simulink model "fft_overlap_tomori"  (R2023b)
settings: Solver=VariableStepAuto  StartTime=0.0  StopTime=inf  RelTol=1e-3
InitFcn:
  | fftparrallelout
  | load('dataram.mat')
  | s= fi(exp(-1j*2*pi.*(0:63)/64),1,16,15);
  | fixed_point = fixdt(1,27,20);
  | fixed_pointu = fixdt(0,29,20);
  | fixed = fixdt(1,22,15);
  | const = fixdt(1,18,17);
  | addConst = fixdt(1,18,16);
  | f =10.4e6;
  | f1=45e6;
  | alpha1 =5;
  | beta1 = 0.00001 ;
  | beta2 = 0.99999 ;
  | beta3 = 23;
undefined symbols (not defined in the file or in its folder): j
libraries: dspxfrm3 x11, commrflib2 x4
(part 2 of 10)

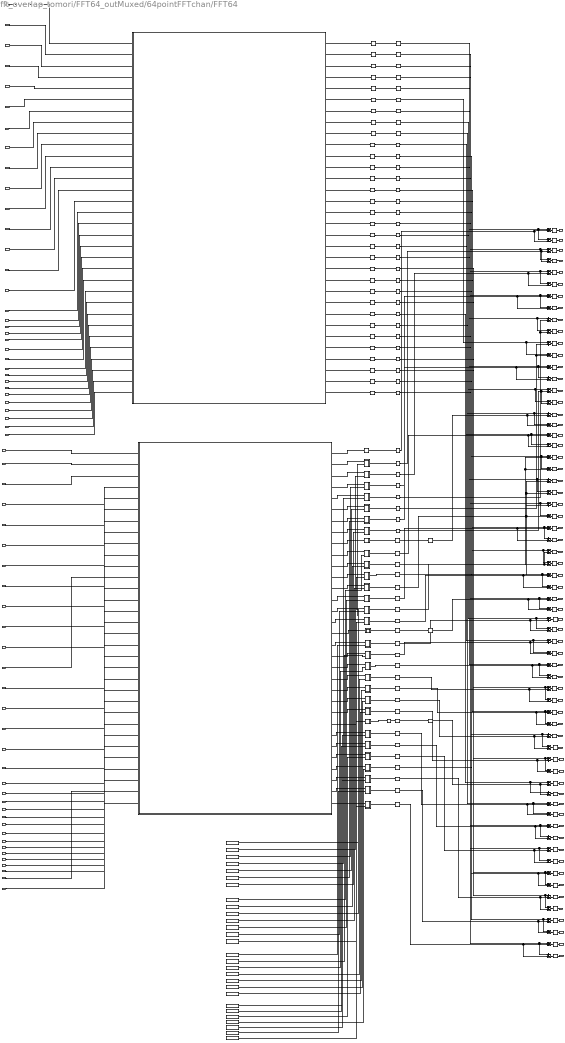
== system fft_overlap_tomori/FFT64_outMuxed/64pointFFTchan/FFT64 ==
  In1 : Inport
  In2 : Inport  Port=2
  In3 : Inport  Port=3
  In4 : Inport  Port=4
  In5 : Inport  Port=5
  In6 : Inport  Port=6
  In7 : Inport  Port=7
  In8 : Inport  Port=8
  In9 : Inport  Port=9
  In10 : Inport  Port=10
  In11 : Inport  Port=11
  In12 : Inport  Port=12
  In13 : Inport  Port=13
  In14 : Inport  Port=14
  In15 : Inport  Port=15
  In17 : Inport  Port=16
  In19 : Inport  Port=17
  In16 : Inport  Port=18
  In18 : Inport  Port=19
  In20 : Inport  Port=20
  In21 : Inport  Port=21
  In22 : Inport  Port=22
  In23 : Inport  Port=23
  In24 : Inport  Port=24
  In25 : Inport  Port=25
  In26 : Inport  Port=26
  In27 : Inport  Port=27
  In28 : Inport  Port=28
  In29 : Inport  Port=29
  In30 : Inport  Port=30
  In31 : Inport  Port=31
  In32 : Inport  Port=32
  In33 : Inport  Port=33
  In34 : Inport  Port=34
  In35 : Inport  Port=35
  In36 : Inport  Port=36
  In37 : Inport  Port=37
  In38 : Inport  Port=38
  In39 : Inport  Port=39
  In40 : Inport  Port=40
  In41 : Inport  Port=41
  In42 : Inport  Port=42
  In43 : Inport  Port=43
  In44 : Inport  Port=44
  In45 : Inport  Port=45
  In46 : Inport  Port=46
  In47 : Inport  Port=47
  In48 : Inport  Port=48
  In49 : Inport  Port=49
  In50 : Inport  Port=50
  In51 : Inport  Port=51
  In52 : Inport  Port=52
  In53 : Inport  Port=53
  In54 : Inport  Port=54
  In55 : Inport  Port=55
  In56 : Inport  Port=56
  In57 : Inport  Port=57
  In58 : Inport  Port=58
  In59 : Inport  Port=59
  In60 : Inport  Port=60
  In61 : Inport  Port=61
  In62 : Inport  Port=62
  In63 : Inport  Port=63
  In64 : Inport  Port=64
  Add{,2,4,6,8,10,12,14,16,18,20,22,24,26,28,30,32,34,36,38,40,42,44..45,47,49,51,53,56,58,60,62} (32 alike) : Sum  OutDataTypeStr=fixed  RndMeth=Round
  Add{1,3,5,7,9,11,13,15,17,19,21,23,25,27,29,31,33,35,37,39,41,43,46,48,50,52,54..55,57,59,61,63} (32 alike) : Sum  Inputs=+-  OutDataTypeStr=fixed  RndMeth=Round
  Constant1 : Constant  Value=exp(-1j*pi/8)  OutDataTypeStr=const  SampleTime=-1
  Constant10 : Constant  Value=exp(-1j*pi*13/16)  OutDataTypeStr=const  SampleTime=-1
  Constant11 : Constant  Value=exp(-1j*pi/32)  OutDataTypeStr=const  SampleTime=-1
  Constant12 : Constant  Value=exp(-1j*7*pi/8)  OutDataTypeStr=const  SampleTime=-1
  Constant13 : Constant  Value=exp(-1j*pi*15/16)  OutDataTypeStr=const  SampleTime=-1
  Constant14 : Constant  Value=exp(-1j*3*pi/32)  OutDataTypeStr=const  SampleTime=-1
  Constant15 : Constant  Value=exp(-1j*pi*3/16)  OutDataTypeStr=const  SampleTime=-1
  Constant16 : Constant  Value=exp(-1j*pi*7/32)  OutDataTypeStr=const  SampleTime=-1
  Constant17 : Constant  Value=exp(-1j*pi*9/32)  OutDataTypeStr=const  SampleTime=-1
  Constant18 : Constant  Value=exp(-1j*pi*11/32)  OutDataTypeStr=const  SampleTime=-1
  Constant19 : Constant  Value=exp(-1j*pi*13/32)  OutDataTypeStr=const  SampleTime=-1
  Constant2 : Constant  Value=exp(-1j*pi/16)  OutDataTypeStr=const  SampleTime=-1
  Constant20 : Constant  Value=exp(-1j*pi*15/32)  OutDataTypeStr=const  SampleTime=-1
  Constant21 : Constant  Value=exp(-1j*pi*17/32)  OutDataTypeStr=const  SampleTime=-1
  Constant22 : Constant  Value=exp(-1j*pi*19/32)  OutDataTypeStr=const  SampleTime=-1
  Constant23 : Constant  Value=exp(-1j*pi*21/32)  OutDataTypeStr=const  SampleTime=-1
  Constant24 : Constant  Value=exp(-1j*pi*23/32)  OutDataTypeStr=const  SampleTime=-1
  Constant25 : Constant  Value=exp(-1j*pi*25/32)  OutDataTypeStr=const  SampleTime=-1
  Constant26 : Constant  Value=exp(-1j*pi*27/32)  OutDataTypeStr=const  SampleTime=-1
  Constant27 : Constant  Value=exp(-1j*pi*29/32)  OutDataTypeStr=const  SampleTime=-1
  Constant28 : Constant  Value=exp(-1j*pi*31/32)  OutDataTypeStr=const  SampleTime=-1
  Constant3 : Constant  Value=exp(-1j*pi*5/32)  OutDataTypeStr=const  SampleTime=-1
  Constant4 : Constant  Value=exp(-1j*pi*5/16)  OutDataTypeStr=const  SampleTime=-1
  Constant5 : Constant  Value=exp(-1j*pi*3/8)  OutDataTypeStr=const  SampleTime=-1
  Constant6 : Constant  Value=exp(-1j*pi*5/8)  OutDataTypeStr=const  SampleTime=-1
  Constant7 : Constant  Value=exp(-1j*pi*7/16)  OutDataTypeStr=const  SampleTime=-1
  Constant8 : Constant  Value=exp(-1j*pi*9/16)  OutDataTypeStr=const  SampleTime=-1
  Constant9 : Constant  Value=exp(-1j*pi*11/16)  OutDataTypeStr=const  SampleTime=-1
  Delay{,9..15,17,20..21,27..32,50..51,53..59,61..98,133..147,149..163} (94 alike) : Delay  DelayLength=1
  Delay{1..8,16,18..19,22..26,33..49,52,60,99..132,164} (70 alike) : Delay  DelayLength=3
  FFT32 : Subsystem
  FFT32_1 : Subsystem
  complexmult : Subsystem
  complexmult1 : Subsystem
  complexmult10 : Subsystem
  complexmult11 : Subsystem
  complexmult12 : Subsystem
  complexmult13 : Subsystem
  complexmult14 : Subsystem
  complexmult15 : Subsystem
  complexmult16 : Subsystem
  complexmult17 : Subsystem
  complexmult18 : Subsystem
  complexmult19 : Subsystem
  complexmult2 : Subsystem
  complexmult20 : Subsystem
  complexmult21 : Subsystem
  complexmult22 : Subsystem
  complexmult23 : Subsystem
  complexmult24 : Subsystem
  complexmult25 : Subsystem
  complexmult26 : Subsystem
  complexmult27 : Subsystem
  complexmult3 : Subsystem
  complexmult4 : Subsystem
  complexmult5 : Subsystem
  complexmult6 : Subsystem
  complexmult7 : Subsystem
  complexmult8 : Subsystem
  complexmult9 : Subsystem
  multByExp(-j*Pi/4) : Subsystem
  multByExp(-j*Pi/4)1 : Subsystem
  multByMinusJ : Subsystem
  multByMinusJ3 : Subsystem
  Out1 : Outport  VectorParamsAs1DForOutWhenUnconnected=off
  Out2 : Outport  Port=2  VectorParamsAs1DForOutWhenUnconnected=off
  Out4 : Outport  Port=3  VectorParamsAs1DForOutWhenUnconnected=off
  Out3 : Outport  Port=4  VectorParamsAs1DForOutWhenUnconnected=off
  Out5 : Outport  Port=5  VectorParamsAs1DForOutWhenUnconnected=off
  Out6 : Outport  Port=6  VectorParamsAs1DForOutWhenUnconnected=off
  Out7 : Outport  Port=7  VectorParamsAs1DForOutWhenUnconnected=off
  Out8 : Outport  Port=8  VectorParamsAs1DForOutWhenUnconnected=off
  Out9 : Outport  Port=9  VectorParamsAs1DForOutWhenUnconnected=off
  Out10 : Outport  Port=10  VectorParamsAs1DForOutWhenUnconnected=off
  Out11 : Outport  Port=11  VectorParamsAs1DForOutWhenUnconnected=off
  Out12 : Outport  Port=12  VectorParamsAs1DForOutWhenUnconnected=off
  Out13 : Outport  Port=13  VectorParamsAs1DForOutWhenUnconnected=off
  Out14 : Outport  Port=14  VectorParamsAs1DForOutWhenUnconnected=off
  Out15 : Outport  Port=15  VectorParamsAs1DForOutWhenUnconnected=off
  Out16 : Outport  Port=16  VectorParamsAs1DForOutWhenUnconnected=off
  Out17 : Outport  Port=17  VectorParamsAs1DForOutWhenUnconnected=off
  Out18 : Outport  Port=18  VectorParamsAs1DForOutWhenUnconnected=off
  Out19 : Outport  Port=19  VectorParamsAs1DForOutWhenUnconnected=off
  Out20 : Outport  Port=20  VectorParamsAs1DForOutWhenUnconnected=off
  Out21 : Outport  Port=21  VectorParamsAs1DForOutWhenUnconnected=off
  Out22 : Outport  Port=22  VectorParamsAs1DForOutWhenUnconnected=off
  Out23 : Outport  Port=23  VectorParamsAs1DForOutWhenUnconnected=off
  Out24 : Outport  Port=24  VectorParamsAs1DForOutWhenUnconnected=off
  Out25 : Outport  Port=25  VectorParamsAs1DForOutWhenUnconnected=off
  Out26 : Outport  Port=26  VectorParamsAs1DForOutWhenUnconnected=off
  Out27 : Outport  Port=27  VectorParamsAs1DForOutWhenUnconnected=off
  Out28 : Outport  Port=28  VectorParamsAs1DForOutWhenUnconnected=off
  Out29 : Outport  Port=29  VectorParamsAs1DForOutWhenUnconnected=off
  Out30 : Outport  Port=30  VectorParamsAs1DForOutWhenUnconnected=off
  Out31 : Outport  Port=31  VectorParamsAs1DForOutWhenUnconnected=off
  Out32 : Outport  Port=32  VectorParamsAs1DForOutWhenUnconnected=off
  Out33 : Outport  Port=33  VectorParamsAs1DForOutWhenUnconnected=off
  Out34 : Outport  Port=34  VectorParamsAs1DForOutWhenUnconnected=off
  Out35 : Outport  Port=35  VectorParamsAs1DForOutWhenUnconnected=off
  Out36 : Outport  Port=36  VectorParamsAs1DForOutWhenUnconnected=off
  Out37 : Outport  Port=37  VectorParamsAs1DForOutWhenUnconnected=off
  Out38 : Outport  Port=38  VectorParamsAs1DForOutWhenUnconnected=off
  Out39 : Outport  Port=39  VectorParamsAs1DForOutWhenUnconnected=off
  Out40 : Outport  Port=40  VectorParamsAs1DForOutWhenUnconnected=off
  Out41 : Outport  Port=41  VectorParamsAs1DForOutWhenUnconnected=off
  Out42 : Outport  Port=42  VectorParamsAs1DForOutWhenUnconnected=off
  Out43 : Outport  Port=43  VectorParamsAs1DForOutWhenUnconnected=off
  Out44 : Outport  Port=44  VectorParamsAs1DForOutWhenUnconnected=off
  Out45 : Outport  Port=45  VectorParamsAs1DForOutWhenUnconnected=off
  Out46 : Outport  Port=46  VectorParamsAs1DForOutWhenUnconnected=off
  Out47 : Outport  Port=47  VectorParamsAs1DForOutWhenUnconnected=off
  Out48 : Outport  Port=48  VectorParamsAs1DForOutWhenUnconnected=off
  Out49 : Outport  Port=49  VectorParamsAs1DForOutWhenUnconnected=off
  Out50 : Outport  Port=50  VectorParamsAs1DForOutWhenUnconnected=off
  Out51 : Outport  Port=51  VectorParamsAs1DForOutWhenUnconnected=off
  Out52 : Outport  Port=52  VectorParamsAs1DForOutWhenUnconnected=off
  Out53 : Outport  Port=53  VectorParamsAs1DForOutWhenUnconnected=off
  Out54 : Outport  Port=54  VectorParamsAs1DForOutWhenUnconnected=off
  Out55 : Outport  Port=55  VectorParamsAs1DForOutWhenUnconnected=off
  Out56 : Outport  Port=56  VectorParamsAs1DForOutWhenUnconnected=off
  Out57 : Outport  Port=57  VectorParamsAs1DForOutWhenUnconnected=off
  Out58 : Outport  Port=58  VectorParamsAs1DForOutWhenUnconnected=off
  Out59 : Outport  Port=59  VectorParamsAs1DForOutWhenUnconnected=off
  Out60 : Outport  Port=60  VectorParamsAs1DForOutWhenUnconnected=off
  Out61 : Outport  Port=61  VectorParamsAs1DForOutWhenUnconnected=off
  Out62 : Outport  Port=62  VectorParamsAs1DForOutWhenUnconnected=off
  Out63 : Outport  Port=63  VectorParamsAs1DForOutWhenUnconnected=off
  Out64 : Outport  Port=64  VectorParamsAs1DForOutWhenUnconnected=off
  wires:
  In13/1 -> FFT32/7(In7)
  In15/1 -> FFT32/8(In8)
  In11/1 -> FFT32/6(In6)
  In19/1 -> FFT32/9(In9)
  In9/1 -> FFT32/5(In5)
  In18/1 -> FFT32/10(In10)
  In7/1 -> FFT32/4(In4)
  In21/1 -> FFT32/11(In11)
  In5/1 -> FFT32/3(In3)
  In23/1 -> FFT32/12(In12)
  In3/1 -> FFT32/2(In2)
  In25/1 -> FFT32/13(In13)
  In1/1 -> FFT32/1(In1)
  In27/1 -> FFT32/14(In14)
  In29/1 -> FFT32/15(In15)
  In31/1 -> FFT32/16(In17)
  In33/1 -> FFT32/17(In19)
  In63/1 -> FFT32/32(In32)
  In61/1 -> FFT32/31(In31)
  In59/1 -> FFT32/30(In30)
  In57/1 -> FFT32/29(In29)
  In55/1 -> FFT32/28(In28)
  In53/1 -> FFT32/27(In27)
  In51/1 -> FFT32/26(In26)
  In49/1 -> FFT32/25(In25)
  In47/1 -> FFT32/24(In24)
  In45/1 -> FFT32/23(In23)
  In43/1 -> FFT32/22(In22)
  In41/1 -> FFT32/21(In21)
  In39/1 -> FFT32/20(In20)
  In37/1 -> FFT32/19(In18)
  In35/1 -> FFT32/18(In16)
  In12/1 -> FFT32_1/6(In6)
  In14/1 -> FFT32_1/7(In7)
  In10/1 -> FFT32_1/5(In5)
  In17/1 -> FFT32_1/8(In8)
  In8/1 -> FFT32_1/4(In4)
  In16/1 -> FFT32_1/9(In9)
  In6/1 -> FFT32_1/3(In3)
  In20/1 -> FFT32_1/10(In10)
  In4/1 -> FFT32_1/2(In2)
  In2/1 -> FFT32_1/1(In1)
  In22/1 -> FFT32_1/11(In11)
  In64/1 -> FFT32_1/32(In32)
  In62/1 -> FFT32_1/31(In31)
  In24/1 -> FFT32_1/12(In12)
  In60/1 -> FFT32_1/30(In30)
  In58/1 -> FFT32_1/29(In29)
  In26/1 -> FFT32_1/13(In13)
  In56/1 -> FFT32_1/28(In28)
  In54/1 -> FFT32_1/27(In27)
  In28/1 -> FFT32_1/14(In14)
  In52/1 -> FFT32_1/26(In26)
  In50/1 -> FFT32_1/25(In25)
  In30/1 -> FFT32_1/15(In15)
  In48/1 -> FFT32_1/24(In24)
  In46/1 -> FFT32_1/23(In23)
  In44/1 -> FFT32_1/22(In22)
  In32/1 -> FFT32_1/16(In17)
  In42/1 -> FFT32_1/21(In21)
  In40/1 -> FFT32_1/20(In20)
  In34/1 -> FFT32_1/17(In19)
  In38/1 -> FFT32_1/19(In18)
  In36/1 -> FFT32_1/18(In16)
  FFT32/1(x0) -> Delay22/1
  FFT32/2(x1) -> Delay18/1
  FFT32/3(x2) -> Delay19/1
  FFT32/4(x3) -> Delay16/1
  FFT32/5(x4) -> Delay23/1
  FFT32/6(x5) -> Delay24/1
  FFT32/7(x6) -> Delay26/1
  FFT32/8(x7) -> Delay33/1
  FFT32/9(x8) -> Delay34/1
  FFT32/10(x9) -> Delay35/1
  FFT32/11(x10) -> Delay37/1
  FFT32/12(x11) -> Delay38/1
  FFT32/13(x12) -> Delay39/1
  FFT32/14(x13) -> Delay36/1
  FFT32/15(x14) -> Delay40/1
  FFT32/16(x15) -> Delay41/1
  FFT32/17(x16) -> Delay42/1
  FFT32/18(x17) -> Delay43/1
  FFT32/19(x18) -> Delay44/1
  FFT32/20(x19) -> Delay45/1
  FFT32/21(x20) -> Delay46/1
  FFT32/22(x21) -> Delay47/1
  FFT32/23(x22) -> Delay48/1
  FFT32/24(x23) -> Delay49/1
  FFT32/25(x24) -> Delay1/1
  FFT32/26(x25) -> Delay2/1
  FFT32/27(x26) -> Delay3/1
  FFT32/28(x27) -> Delay4/1
  FFT32/29(x28) -> Delay5/1
  FFT32/30(x29) -> Delay6/1
  FFT32/31(x30) -> Delay7/1
  FFT32/32(x31) -> Delay8/1
  FFT32_1/25(x24) -> multByExp(-j*Pi/4)1/1(x4)
  Delay22/1 -> Delay105/1
  Delay18/1 -> Delay102/1
  Delay19/1 -> Delay103/1
  Delay16/1 -> Delay101/1
  Delay23/1 -> Delay106/1
  Delay24/1 -> Delay107/1
  Delay26/1 -> Delay108/1
  Delay33/1 -> Delay110/1
  Delay34/1 -> Delay111/1
  Delay35/1 -> Delay112/1
  Delay37/1 -> Delay114/1
  Delay38/1 -> Delay115/1
  Delay39/1 -> Delay116/1
  Delay36/1 -> Delay113/1
  Delay40/1 -> Delay118/1
  Delay41/1 -> Delay119/1
  Delay42/1 -> Delay120/1
  Delay43/1 -> Delay121/1
  Delay44/1 -> Delay122/1
  Delay45/1 -> Delay123/1
  Delay46/1 -> Delay124/1
  Delay47/1 -> Delay125/1
  Delay48/1 -> Delay126/1
  Delay49/1 -> Delay127/1
  Delay1/1 -> Delay100/1
  Delay2/1 -> Delay104/1
  Delay3/1 -> Delay109/1
  Delay4/1 -> Delay117/1
  Delay5/1 -> Delay128/1
  Delay6/1 -> Delay129/1
  Delay7/1 -> Delay130/1
  Delay8/1 -> Delay131/1
  FFT32_1/1(x0) -> Delay99/1
  Add4/1 -> Delay17/1
  Add/1 -> Delay/1
  Add2/1 -> Delay66/1
  Add6/1 -> Delay20/1
  Add8/1 -> Delay21/1
  Add10/1 -> Delay9/1
  Add12/1 -> Delay12/1
  Add14/1 -> Delay13/1
  Add16/1 -> Delay32/1
  Add24/1 -> Delay65/1
  Add26/1 -> Delay56/1
  Add28/1 -> Delay57/1
  Add30/1 -> Delay58/1
  Add18/1 -> Delay59/1
  Add20/1 -> Delay51/1
  Add22/1 -> Delay53/1
  Add32/1 -> Delay67/1
  Add44/1 -> Delay97/1
  Add58/1 -> Delay74/1
  Add60/1 -> Delay75/1
  Add62/1 -> Delay76/1
  Add34/1 -> Delay98/1
  Add36/1 -> Delay70/1
  Add38/1 -> Delay71/1
  Add40/1 -> Delay82/1
  Add49/1 -> Delay96/1
  Add51/1 -> Delay88/1
  Add53/1 -> Delay89/1
  Add56/1 -> Delay90/1
  Add42/1 -> Delay91/1
  Add45/1 -> Delay84/1
  Add47/1 -> Delay85/1
  Add1/1 -> Delay28/1
  Add3/1 -> Delay29/1
  Add5/1 -> Delay30/1
  Add7/1 -> Delay31/1
  Add9/1 -> Delay10/1
  Add11/1 -> Delay11/1
  Add13/1 -> Delay14/1
  Add15/1 -> Delay15/1
  Add17/1 -> Delay61/1
  Add25/1 -> Delay62/1
  Add27/1 -> Delay63/1
  Add29/1 -> Delay64/1
  Add31/1 -> Delay27/1
  Add19/1 -> Delay50/1
  Add21/1 -> Delay54/1
  Add23/1 -> Delay55/1
  Add33/1 -> Delay78/1
  Add55/1 -> Delay79/1
  Add59/1 -> Delay80/1
  Add61/1 -> Delay81/1
  Add63/1 -> Delay68/1
  Add35/1 -> Delay69/1
  Add37/1 -> Delay72/1
  Add39/1 -> Delay73/1
  Add41/1 -> Delay92/1
  Add50/1 -> Delay93/1
  Add52/1 -> Delay94/1
  Add54/1 -> Delay95/1
  Add57/1 -> Delay77/1
  Add43/1 -> Delay83/1
  Add46/1 -> Delay86/1
  Add48/1 -> Delay87/1
  FFT32_1/2(x1) -> complexmult/1(x1)
  Constant11/1 -> complexmult/2(In3)
  complexmult/1(Out1) -> Delay133/1
  FFT32_1/3(x2) -> complexmult1/1(x1)
  Constant2/1 -> complexmult1/2(In3)
  FFT32_1/4(x3) -> complexmult2/1(x1)
  Constant14/1 -> complexmult2/2(In3)
  FFT32_1/5(x4) -> complexmult3/1(x1)
  Constant1/1 -> complexmult3/2(In3)
  FFT32_1/6(x5) -> complexmult4/1(x1)
  Constant3/1 -> complexmult4/2(In3)
  FFT32_1/7(x6) -> complexmult5/1(x1)
  multByExp(-j*Pi/4)/1(Out1) -> Delay140/1
  FFT32_1/10(x9) -> complexmult7/1(x1)
  Constant15/1 -> complexmult5/2(In3)
  FFT32_1/9(x8) -> multByExp(-j*Pi/4)/1(x4)
  FFT32_1/8(x7) -> complexmult6/1(x1)
  Constant16/1 -> complexmult6/2(In3)
  Constant17/1 -> complexmult7/2(In3)
  FFT32_1/11(x10) -> complexmult8/1(x1)
  Constant4/1 -> complexmult8/2(In3)
  FFT32_1/12(x11) -> complexmult9/1(x1)
  Constant18/1 -> complexmult9/2(In3)
  FFT32_1/13(x12) -> complexmult10/1(x1)
  Constant5/1 -> complexmult10/2(In3)
  FFT32_1/14(x13) -> complexmult11/1(x1)
  FFT32_1/15(x14) -> complexmult12/1(x1)
  Constant7/1 -> complexmult12/2(In3)
  FFT32_1/16(x15) -> complexmult13/1(x1)
  Constant20/1 -> complexmult13/2(In3)
  FFT32_1/17(x16) -> multByMinusJ/1(x4)
  multByMinusJ/1(Out1) -> Delay25/1
  FFT32_1/18(x17) -> complexmult14/1(x1)
  Constant21/1 -> complexmult14/2(In3)
  FFT32_1/19(x18) -> complexmult15/1(x1)
  FFT32_1/20(x19) -> complexmult16/1(x1)
  FFT32_1/21(x20) -> complexmult17/1(x1)
  FFT32_1/22(x21) -> complexmult18/1(x1)
  FFT32_1/23(x22) -> complexmult19/1(x1)
  Constant19/1 -> complexmult11/2(In3)
  Constant8/1 -> complexmult15/2(In3)
  Constant22/1 -> complexmult16/2(In3)
  Constant6/1 -> complexmult17/2(In3)
  Constant23/1 -> complexmult18/2(In3)
  Constant9/1 -> complexmult19/2(In3)
  FFT32_1/24(x23) -> complexmult20/1(x1)
  Constant24/1 -> complexmult20/2(In3)
  multByMinusJ3/1(Out1) -> Delay156/1
  multByExp(-j*Pi/4)1/1(Out1) -> multByMinusJ3/1(In1)
  FFT32_1/26(x25) -> complexmult21/1(x1)
  FFT32_1/27(x26) -> complexmult22/1(x1)
  FFT32_1/28(x27) -> complexmult23/1(x1)
  FFT32_1/29(x28) -> complexmult24/1(x1)
  FFT32_1/30(x29) -> complexmult25/1(x1)
  FFT32_1/32(x31) -> complexmult27/1(x1)
  FFT32_1/31(x30) -> complexmult26/1(x1)
  Constant25/1 -> complexmult21/2(In3)
  Constant10/1 -> complexmult22/2(In3)
  Constant26/1 -> complexmult23/2(In3)
  Constant12/1 -> complexmult24/2(In3)
  Constant27/1 -> complexmult25/2(In3)
  Constant13/1 -> complexmult26/2(In3)
  Constant28/1 -> complexmult27/2(In3)
  Delay82/1 -> Out25/1
  Delay83/1 -> Out62/1
  Delay84/1 -> Out31/1
  Delay85/1 -> Out32/1
  Delay86/1 -> Out63/1
  Delay77/1 -> Out61/1
  Delay73/1 -> Out56/1
  Delay71/1 -> Out24/1
  Delay91/1 -> Out30/1
  Delay92/1 -> Out57/1
  Delay93/1 -> Out58/1
  Delay94/1 -> Out59/1
  Delay95/1 -> Out60/1
  Delay96/1 -> Out26/1
  Delay87/1 -> Out64/1
  Delay88/1 -> Out27/1
  Delay89/1 -> Out28/1
  Delay90/1 -> Out29/1
  Delay72/1 -> Out55/1
  Delay70/1 -> Out23/1
  Delay69/1 -> Out54/1
  Delay98/1 -> Out22/1
  Delay68/1 -> Out53/1
  Delay76/1 -> Out21/1
  Delay81/1 -> Out52/1
  Delay75/1 -> Out20/1
  Delay74/1 -> Out19/1
  Delay80/1 -> Out51/1
  Delay79/1 -> Out50/1
  Delay97/1 -> Out18/1
  Delay78/1 -> Out49/1
  Delay67/1 -> Out17/1
  Delay50/1 -> Out46/1
  Delay28/1 -> Out33/1
  Delay14/1 -> Out39/1
  Delay17/1 -> Out4/1
  Delay12/1 -> Out7/1
  Delay54/1 -> Out47/1
  Delay10/1 -> Out37/1
  Delay59/1 -> Out14/1
  Delay51/1 -> Out15/1
  Delay21/1 -> Out5/1
  Delay/1 -> Out1/1
  Delay11/1 -> Out38/1
  Delay55/1 -> Out48/1
  Delay13/1 -> Out8/1
  Delay31/1 -> Out36/1
  Delay27/1 -> Out45/1
  Delay9/1 -> Out6/1
  Delay66/1 -> Out2/1
  Delay30/1 -> Out35/1
  Delay53/1 -> Out16/1
  Delay29/1 -> Out34/1
  Delay20/1 -> Out3/1
  Delay58/1 -> Out13/1
  Delay64/1 -> Out44/1
  Delay57/1 -> Out12/1
  Delay63/1 -> Out43/1
  Delay56/1 -> Out11/1
  Delay62/1 -> Out42/1
  Delay65/1 -> Out10/1
  Delay61/1 -> Out41/1
  Delay32/1 -> Out9/1
  Delay15/1 -> Out40/1
  complexmult1/1(Out1) -> Delay134/1
  complexmult2/1(Out1) -> Delay135/1
  complexmult3/1(Out1) -> Delay136/1
  complexmult4/1(Out1) -> Delay137/1
  complexmult5/1(Out1) -> Delay138/1
  complexmult6/1(Out1) -> Delay139/1
  Delay132/1 -> Add17/2, Add16/2
  complexmult7/1(Out1) -> Delay141/1
  complexmult8/1(Out1) -> Delay142/1
  complexmult9/1(Out1) -> Delay143/1
  complexmult10/1(Out1) -> Delay144/1
  complexmult11/1(Out1) -> Delay145/1
  complexmult12/1(Out1) -> Delay146/1
  complexmult13/1(Out1) -> Delay147/1
  Delay52/1 -> Add33/2, Add32/2
  complexmult14/1(Out1) -> Delay149/1
  complexmult15/1(Out1) -> Delay150/1
  complexmult16/1(Out1) -> Delay151/1
  complexmult17/1(Out1) -> Delay152/1
  complexmult18/1(Out1) -> Delay153/1
  complexmult19/1(Out1) -> Delay154/1
  complexmult20/1(Out1) -> Delay155/1
  Delay60/1 -> Add41/2, Add40/2
  complexmult21/1(Out1) -> Delay157/1
  complexmult22/1(Out1) -> Delay158/1
  complexmult23/1(Out1) -> Delay159/1
  complexmult24/1(Out1) -> Delay160/1
  complexmult25/1(Out1) -> Delay161/1
  complexmult26/1(Out1) -> Delay162/1
  complexmult27/1(Out1) -> Delay163/1
  Delay99/1 -> Delay164/1
  Delay105/1 -> Add1/1, Add/1
  Delay102/1 -> Add3/1, Add2/1
  Delay103/1 -> Add5/1, Add4/1
  Delay101/1 -> Add6/1, Add7/1
  Delay106/1 -> Add9/1, Add8/1
  Delay107/1 -> Add11/1, Add10/1
  Delay108/1 -> Add13/1, Add12/1
  Delay110/1 -> Add15/1, Add14/1
  Delay111/1 -> Add17/1, Add16/1
  Delay112/1 -> Add24/1, Add25/1
  Delay114/1 -> Add27/1, Add26/1
  Delay115/1 -> Add29/1, Add28/1
  Delay116/1 -> Add31/1, Add30/1
  Delay113/1 -> Add19/1, Add18/1
  Delay118/1 -> Add21/1, Add20/1
  Delay119/1 -> Add23/1, Add22/1
  Delay120/1 -> Add33/1, Add32/1
  Delay121/1 -> Add55/1, Add44/1
  Delay122/1 -> Add59/1, Add58/1
  Delay123/1 -> Add61/1, Add60/1
  Delay124/1 -> Add63/1, Add62/1
  Delay125/1 -> Add35/1, Add34/1
  Delay126/1 -> Add37/1, Add36/1
  Delay127/1 -> Add39/1, Add38/1
  Delay100/1 -> Add40/1, Add41/1
  Delay104/1 -> Add50/1, Add49/1
  Delay109/1 -> Add52/1, Add51/1
  Delay117/1 -> Add54/1, Add53/1
  Delay128/1 -> Add57/1, Add56/1
  Delay129/1 -> Add43/1, Add42/1
  Delay130/1 -> Add46/1, Add45/1
  Delay131/1 -> Add48/1, Add47/1
  Delay164/1 -> Add/2, Add1/2
  Delay133/1 -> Add3/2, Add2/2
  Delay134/1 -> Add5/2, Add4/2
  Delay135/1 -> Add7/2, Add6/2
  Delay136/1 -> Add8/2, Add9/2
  Delay137/1 -> Add10/2, Add11/2
  Delay138/1 -> Add13/2, Add12/2
  Delay139/1 -> Add15/2, Add14/2
  Delay140/1 -> Delay132/1
  Delay141/1 -> Add25/2, Add24/2
  Delay142/1 -> Add26/2, Add27/2
  Delay143/1 -> Add28/2, Add29/2
  Delay144/1 -> Add30/2, Add31/2
  Delay145/1 -> Add19/2, Add18/2
  Delay146/1 -> Add20/2, Add21/2
  Delay147/1 -> Add23/2, Add22/2
  Delay25/1 -> Delay52/1
  Delay149/1 -> Add55/2, Add44/2
  Delay150/1 -> Add59/2, Add58/2
  Delay151/1 -> Add61/2, Add60/2
  Delay152/1 -> Add63/2, Add62/2
  Delay153/1 -> Add35/2, Add34/2
  Delay154/1 -> Add37/2, Add36/2
  Delay155/1 -> Add39/2, Add38/2
  Delay156/1 -> Delay60/1
  Delay157/1 -> Add50/2, Add49/2
  Delay158/1 -> Add52/2, Add51/2
  Delay159/1 -> Add54/2, Add53/2
  Delay160/1 -> Add57/2, Add56/2
  Delay161/1 -> Add43/2, Add42/2
  Delay162/1 -> Add46/2, Add45/2
  Delay163/1 -> Add48/2, Add47/2

== system fft_overlap_tomori/16//32 and test junk/16/FFT16/FFT8 ==
  In1 : Inport
  In2 : Inport  Port=2
  In3 : Inport  Port=3
  In4 : Inport  Port=4
  In5 : Inport  Port=5
  In6 : Inport  Port=6
  In7 : Inport  Port=7
  In8 : Inport  Port=8
  Add{,2,4,6,8,10,12,14,16,18,20,22} (12 alike) : Sum  OutDataTypeStr=fixed  RndMeth=Round
  Add{1,3,5,7,9,11,13,15,17,19,21,23} (12 alike) : Sum  Inputs=+-  OutDataTypeStr=fixed  RndMeth=Round
  Delay{,1,4..9,12..13,16..23} (18 alike) : Delay  DelayLength=1
  Delay{2..3,10..11,14..15} (6 alike) : Delay  DelayLength=3
  multByExp(-j*Pi/4) : Subsystem
  multByExp(-j*Pi/4)1 : Subsystem
  multByMinusJ : Subsystem
  multByMinusJ1 : Subsystem
  multByMinusJ2 : Subsystem
  multByMinusJ3 : Subsystem
  x0 : Outport
  x1 : Outport  Port=2  VectorParamsAs1DForOutWhenUnconnected=off
  x2 : Outport  Port=3  VectorParamsAs1DForOutWhenUnconnected=off
  x3 : Outport  Port=4  VectorParamsAs1DForOutWhenUnconnected=off
  x4 : Outport  Port=5  VectorParamsAs1DForOutWhenUnconnected=off
  x5 : Outport  Port=6  VectorParamsAs1DForOutWhenUnconnected=off
  x6 : Outport  Port=7  VectorParamsAs1DForOutWhenUnconnected=off
  x7 : Outport  Port=8  VectorParamsAs1DForOutWhenUnconnected=off
  wires:
  In1/1 -> Add1/1, Add/1
  In5/1 -> Add/2, Add1/2
  Add/1 -> Delay/1
  Add1/1 -> Delay1/1
  Delay/1 -> Add2/1, Add3/1
  Add2/1 -> Delay2/1
  Add3/1 -> Delay3/1
  In3/1 -> Add7/1, Add6/1
  In7/1 -> Add6/2, Add7/2
  In2/1 -> Add5/1, Add4/1
  In6/1 -> Add4/2, Add5/2
  In4/1 -> Add9/1, Add8/1
  In8/1 -> Add8/2, Add9/2
  Add4/1 -> Delay4/1
  Add5/1 -> Delay5/1
  Add6/1 -> Delay6/1
  Add7/1 -> multByMinusJ/1(In1)
  Add8/1 -> Delay8/1
  Add9/1 -> multByMinusJ1/1(In1)
  Delay4/1 -> Add10/1, Add11/1
  Delay8/1 -> Add11/2, Add10/2
  Add10/1 -> Delay10/1
  Add11/1 -> multByMinusJ2/1(In1)
  Delay6/1 -> Add2/2, Add3/2
  Delay2/1 -> Add22/1, Add23/1
  Delay10/1 -> Add23/2, Add22/2
  Add22/1 -> Delay12/1
  Add23/1 -> Delay13/1
  Delay12/1 -> x0/1
  Delay13/1 -> x4/1
  Delay1/1 -> Add14/1, Add15/1
  Delay7/1 -> Add14/2, Add15/2
  Add14/1 -> Delay14/1
  Add15/1 -> Delay15/1
  multByMinusJ/1(Out1) -> Delay7/1
  multByMinusJ1/1(Out1) -> Delay9/1
  Delay5/1 -> Add17/1, Add16/1
  Delay9/1 -> Add17/2, Add16/2
  Add16/1 -> multByExp(-j*Pi/4)/1(In1)
  Add17/1 -> multByExp(-j*Pi/4)1/1(In1)
  Delay3/1 -> Add13/1, Add12/1
  Add12/1 -> Delay18/1
  Add13/1 -> Delay19/1
  multByMinusJ2/1(Out1) -> Delay11/1
  Delay11/1 -> Add13/2, Add12/2
  Delay18/1 -> x2/1
  Delay19/1 -> x6/1
  Add18/1 -> Delay20/1
  Add19/1 -> Delay21/1
  Add20/1 -> Delay22/1
  Add21/1 -> Delay23/1
  Delay14/1 -> Add18/1, Add19/1
  Delay16/1 -> Add19/2, Add18/2
  multByMinusJ3/1(Out1) -> Delay17/1
  multByExp(-j*Pi/4)/1(Out1) -> Delay16/1
  multByExp(-j*Pi/4)1/1(Out1) -> multByMinusJ3/1(In1)
  Delay20/1 -> x1/1
  Delay21/1 -> x5/1
  Delay22/1 -> x3/1
  Delay23/1 -> x7/1
  Delay15/1 -> Add20/1, Add21/1
  Delay17/1 -> Add20/2, Add21/2

== system fft_overlap_tomori/16//32 and test junk/16/FFT16/FFT8_1 ==
  In1 : Inport
  In2 : Inport  Port=2
  In3 : Inport  Port=3
  In4 : Inport  Port=4
  In5 : Inport  Port=5
  In6 : Inport  Port=6
  In7 : Inport  Port=7
  In8 : Inport  Port=8
  Add{,2,4,6,8,10,12,14,16,18,20,22} (12 alike) : Sum  OutDataTypeStr=fixed  RndMeth=Round
  Add{1,3,5,7,9,11,13,15,17,19,21,23} (12 alike) : Sum  Inputs=+-  OutDataTypeStr=fixed  RndMeth=Round
  Delay{,1,4..9,12..13,16..23} (18 alike) : Delay  DelayLength=1
  Delay{2..3,10..11,14..15} (6 alike) : Delay  DelayLength=3
  multByExp(-j*Pi/4) : Subsystem
  multByExp(-j*Pi/4)1 : Subsystem
  multByMinusJ : Subsystem
  multByMinusJ1 : Subsystem
  multByMinusJ2 : Subsystem
  multByMinusJ3 : Subsystem
  x0 : Outport
  x1 : Outport  Port=2  VectorParamsAs1DForOutWhenUnconnected=off
  x2 : Outport  Port=3  VectorParamsAs1DForOutWhenUnconnected=off
  x3 : Outport  Port=4  VectorParamsAs1DForOutWhenUnconnected=off
  x4 : Outport  Port=5  VectorParamsAs1DForOutWhenUnconnected=off
  x5 : Outport  Port=6  VectorParamsAs1DForOutWhenUnconnected=off
  x6 : Outport  Port=7  VectorParamsAs1DForOutWhenUnconnected=off
  x7 : Outport  Port=8  VectorParamsAs1DForOutWhenUnconnected=off
  wires:
  In1/1 -> Add1/1, Add/1
  In5/1 -> Add/2, Add1/2
  Add/1 -> Delay/1
  Add1/1 -> Delay1/1
  Delay/1 -> Add2/1, Add3/1
  Add2/1 -> Delay2/1
  Add3/1 -> Delay3/1
  In3/1 -> Add7/1, Add6/1
  In7/1 -> Add6/2, Add7/2
  In2/1 -> Add5/1, Add4/1
  In6/1 -> Add4/2, Add5/2
  In4/1 -> Add9/1, Add8/1
  In8/1 -> Add8/2, Add9/2
  Add4/1 -> Delay4/1
  Add5/1 -> Delay5/1
  Add6/1 -> Delay6/1
  Add7/1 -> multByMinusJ/1(In1)
  Add8/1 -> Delay8/1
  Add9/1 -> multByMinusJ1/1(In1)
  Delay4/1 -> Add10/1, Add11/1
  Delay8/1 -> Add11/2, Add10/2
  Add10/1 -> Delay10/1
  Add11/1 -> multByMinusJ2/1(In1)
  Delay6/1 -> Add2/2, Add3/2
  Delay2/1 -> Add22/1, Add23/1
  Delay10/1 -> Add23/2, Add22/2
  Add22/1 -> Delay12/1
  Add23/1 -> Delay13/1
  Delay12/1 -> x0/1
  Delay13/1 -> x4/1
  Delay1/1 -> Add14/1, Add15/1
  Delay7/1 -> Add14/2, Add15/2
  Add14/1 -> Delay14/1
  Add15/1 -> Delay15/1
  multByMinusJ/1(Out1) -> Delay7/1
  multByMinusJ1/1(Out1) -> Delay9/1
  Delay5/1 -> Add17/1, Add16/1
  Delay9/1 -> Add17/2, Add16/2
  Add16/1 -> multByExp(-j*Pi/4)/1(In1)
  Add17/1 -> multByExp(-j*Pi/4)1/1(In1)
  Delay3/1 -> Add13/1, Add12/1
  Add12/1 -> Delay18/1
  Add13/1 -> Delay19/1
  multByMinusJ2/1(Out1) -> Delay11/1
  Delay11/1 -> Add13/2, Add12/2
  Delay18/1 -> x2/1
  Delay19/1 -> x6/1
  Add18/1 -> Delay20/1
  Add19/1 -> Delay21/1
  Add20/1 -> Delay22/1
  Add21/1 -> Delay23/1
  Delay14/1 -> Add18/1, Add19/1
  Delay16/1 -> Add19/2, Add18/2
  multByMinusJ3/1(Out1) -> Delay17/1
  multByExp(-j*Pi/4)/1(Out1) -> Delay16/1
  multByExp(-j*Pi/4)1/1(Out1) -> multByMinusJ3/1(In1)
  Delay20/1 -> x1/1
  Delay21/1 -> x5/1
  Delay22/1 -> x3/1
  Delay23/1 -> x7/1
  Delay15/1 -> Add20/1, Add21/1
  Delay17/1 -> Add20/2, Add21/2

== system fft_overlap_tomori/16//32 and test junk/16/FFT16/complexmult ==
  x1 : Inport
  In3 : Inport  Port=2
  Add1 : Sum  OutDataTypeStr=fixed  RndMeth=Round
  Add20 : Sum  OutDataTypeStr=fixed  RndMeth=Round
  Add3 : Sum  Inputs=+--  OutDataTypeStr=fixed  AccumDataTypeStr=fixed  RndMeth=Round
  Add4 : Sum  Inputs=+-  OutDataTypeStr=fixed  AccumDataTypeStr=fixed  RndMeth=Round
  Complex to Real-Imag : ComplexToRealImag
  Complex to Real-Imag1 : ComplexToRealImag
  Constant : Constant  Commented=on  Value=1+j  OutDataTypeStr=fixdt(1,22, 15)  SampleTime=2e-8
  Constant1 : Constant  Commented=on  Value=1-j  OutDataTypeStr=fixdt(1,22, 15)  SampleTime=2e-8
  Delay : Delay  DelayLength=3
  Delay1 : Delay  DelayLength=3
  Delay2 : Delay  DelayLength=3
  Display : Display  Commented=on
  Product : Product  OutDataTypeStr=fixed  RndMeth=Round
  Product1 : Product  OutDataTypeStr=fixed  RndMeth=Round
  Product2 : Product  OutDataTypeStr=fixed  RndMeth=Round
  Real-Imag to Complex : RealImagToComplex
  Out1 : Outport
  wires:
  Complex to Real-Imag1/2 -> Add1/2, Product2/2
  Complex to Real-Imag/2 -> Add20/2, Product2/1
  Complex to Real-Imag1/1 -> Add1/1, Product1/2
  Complex to Real-Imag/1 -> Add20/1, Product1/1
  Add1/1 -> Product/2
  Add20/1 -> Product/1
  Add3/1 -> Real-Imag to Complex/2
  Add4/1 -> Real-Imag to Complex/1
  Delay2/1 -> Add4/2, Add3/3
  Delay1/1 -> Add3/2, Add4/1
  Delay/1 -> Add3/1
  Product2/1 -> Delay2/1
  Product1/1 -> Delay1/1
  Product/1 -> Delay/1
  x1/1 -> Complex to Real-Imag/1
  In3/1 -> Complex to Real-Imag1/1
  Real-Imag to Complex/1 -> Out1/1

== system fft_overlap_tomori/16//32 and test junk/16/FFT16/complexmult1 ==
  x1 : Inport
  In3 : Inport  Port=2
  Add1 : Sum  OutDataTypeStr=fixed  RndMeth=Round
  Add20 : Sum  OutDataTypeStr=fixed  RndMeth=Round
  Add3 : Sum  Inputs=+--  OutDataTypeStr=fixed  AccumDataTypeStr=fixed  RndMeth=Round
  Add4 : Sum  Inputs=+-  OutDataTypeStr=fixed  AccumDataTypeStr=fixed  RndMeth=Round
  Complex to Real-Imag : ComplexToRealImag
  Complex to Real-Imag1 : ComplexToRealImag
  Constant : Constant  Commented=on  Value=1+j  OutDataTypeStr=fixdt(1,22, 15)  SampleTime=2e-8
  Constant1 : Constant  Commented=on  Value=1-j  OutDataTypeStr=fixdt(1,22, 15)  SampleTime=2e-8
  Delay : Delay  DelayLength=3
  Delay1 : Delay  DelayLength=3
  Delay2 : Delay  DelayLength=3
  Display : Display  Commented=on
  Product : Product  OutDataTypeStr=fixed  RndMeth=Round
  Product1 : Product  OutDataTypeStr=fixed  RndMeth=Round
  Product2 : Product  OutDataTypeStr=fixed  RndMeth=Round
  Real-Imag to Complex : RealImagToComplex
  Out1 : Outport
  wires:
  Real-Imag to Complex/1 -> Out1/1
  In3/1 -> Complex to Real-Imag1/1
  x1/1 -> Complex to Real-Imag/1
  Product/1 -> Delay/1
  Product1/1 -> Delay1/1
  Product2/1 -> Delay2/1
  Delay/1 -> Add3/1
  Delay1/1 -> Add4/1, Add3/2
  Delay2/1 -> Add3/3, Add4/2
  Add4/1 -> Real-Imag to Complex/1
  Add3/1 -> Real-Imag to Complex/2
  Add20/1 -> Product/1
  Add1/1 -> Product/2
  Complex to Real-Imag/1 -> Product1/1, Add20/1
  Complex to Real-Imag1/1 -> Product1/2, Add1/1
  Complex to Real-Imag/2 -> Product2/1, Add20/2
  Complex to Real-Imag1/2 -> Product2/2, Add1/2

== system fft_overlap_tomori/16//32 and test junk/16/FFT16/complexmult2 ==
  x1 : Inport
  In3 : Inport  Port=2
  Add1 : Sum  OutDataTypeStr=fixed  RndMeth=Round
  Add20 : Sum  OutDataTypeStr=fixed  RndMeth=Round
  Add3 : Sum  Inputs=+--  OutDataTypeStr=fixed  AccumDataTypeStr=fixed  RndMeth=Round
  Add4 : Sum  Inputs=+-  OutDataTypeStr=fixed  AccumDataTypeStr=fixed  RndMeth=Round
  Complex to Real-Imag : ComplexToRealImag
  Complex to Real-Imag1 : ComplexToRealImag
  Constant : Constant  Commented=on  Value=1+j  OutDataTypeStr=fixdt(1,22, 15)  SampleTime=2e-8
  Constant1 : Constant  Commented=on  Value=1-j  OutDataTypeStr=fixdt(1,22, 15)  SampleTime=2e-8
  Delay : Delay  DelayLength=3
  Delay1 : Delay  DelayLength=3
  Delay2 : Delay  DelayLength=3
  Display : Display  Commented=on
  Product : Product  OutDataTypeStr=fixed  RndMeth=Round
  Product1 : Product  OutDataTypeStr=fixed  RndMeth=Round
  Product2 : Product  OutDataTypeStr=fixed  RndMeth=Round
  Real-Imag to Complex : RealImagToComplex
  Out1 : Outport
  wires:
  Complex to Real-Imag1/2 -> Add1/2, Product2/2
  Complex to Real-Imag/2 -> Add20/2, Product2/1
  Complex to Real-Imag1/1 -> Add1/1, Product1/2
  Complex to Real-Imag/1 -> Add20/1, Product1/1
  Add1/1 -> Product/2
  Add20/1 -> Product/1
  Add3/1 -> Real-Imag to Complex/2
  Add4/1 -> Real-Imag to Complex/1
  Delay2/1 -> Add4/2, Add3/3
  Delay1/1 -> Add3/2, Add4/1
  Delay/1 -> Add3/1
  Product2/1 -> Delay2/1
  Product1/1 -> Delay1/1
  Product/1 -> Delay/1
  x1/1 -> Complex to Real-Imag/1
  In3/1 -> Complex to Real-Imag1/1
  Real-Imag to Complex/1 -> Out1/1

== system fft_overlap_tomori/16//32 and test junk/16/FFT16/complexmult3 ==
  x1 : Inport
  In3 : Inport  Port=2
  Add1 : Sum  OutDataTypeStr=fixed  RndMeth=Round
  Add20 : Sum  OutDataTypeStr=fixed  RndMeth=Round
  Add3 : Sum  Inputs=+--  OutDataTypeStr=fixed  AccumDataTypeStr=fixed  RndMeth=Round
  Add4 : Sum  Inputs=+-  OutDataTypeStr=fixed  AccumDataTypeStr=fixed  RndMeth=Round
  Complex to Real-Imag : ComplexToRealImag
  Complex to Real-Imag1 : ComplexToRealImag
  Constant : Constant  Commented=on  Value=1+j  OutDataTypeStr=fixdt(1,22, 15)  SampleTime=2e-8
  Constant1 : Constant  Commented=on  Value=1-j  OutDataTypeStr=fixdt(1,22, 15)  SampleTime=2e-8
  Delay : Delay  DelayLength=3
  Delay1 : Delay  DelayLength=3
  Delay2 : Delay  DelayLength=3
  Display : Display  Commented=on
  Product : Product  OutDataTypeStr=fixed  RndMeth=Round
  Product1 : Product  OutDataTypeStr=fixed  RndMeth=Round
  Product2 : Product  OutDataTypeStr=fixed  RndMeth=Round
  Real-Imag to Complex : RealImagToComplex
  Out1 : Outport
  wires:
  Real-Imag to Complex/1 -> Out1/1
  In3/1 -> Complex to Real-Imag1/1
  x1/1 -> Complex to Real-Imag/1
  Product/1 -> Delay/1
  Product1/1 -> Delay1/1
  Product2/1 -> Delay2/1
  Delay/1 -> Add3/1
  Delay1/1 -> Add4/1, Add3/2
  Delay2/1 -> Add3/3, Add4/2
  Add4/1 -> Real-Imag to Complex/1
  Add3/1 -> Real-Imag to Complex/2
  Add20/1 -> Product/1
  Add1/1 -> Product/2
  Complex to Real-Imag/1 -> Product1/1, Add20/1
  Complex to Real-Imag1/1 -> Product1/2, Add1/1
  Complex to Real-Imag/2 -> Product2/1, Add20/2
  Complex to Real-Imag1/2 -> Product2/2, Add1/2

== system fft_overlap_tomori/16//32 and test junk/16/FFT16/multByExp(-j*Pi//4) ==
  In1 : Inport
  Add : Sum  OutDataTypeStr=fixed  RndMeth=Round
  Add1 : Sum  Inputs=+-  OutDataTypeStr=fixed  RndMeth=Round
  Complex to Real-Imag : ComplexToRealImag
  Delay24 : Delay
  Gain : Gain  Gain=sqrt(2)/2  ParamDataTypeStr=fixed  OutDataTypeStr=fixed  RndMeth=Round
  Real-Imag to Complex : RealImagToComplex
  Out1 : Outport
  wires:
  Gain/1 -> Delay24/1
  Complex to Real-Imag/1 -> Add1/2, Add/1
  Complex to Real-Imag/2 -> Add1/1, Add/2
  Add/1 -> Real-Imag to Complex/1
  Add1/1 -> Real-Imag to Complex/2
  Delay24/1 -> Complex to Real-Imag/1
  Real-Imag to Complex/1 -> Out1/1
  In1/1 -> Gain/1

== system fft_overlap_tomori/16//32 and test junk/16/FFT16/multByExp(-j*Pi//4)1 ==
  In1 : Inport
  Add : Sum  OutDataTypeStr=fixed  RndMeth=Round
  Add1 : Sum  Inputs=+-  OutDataTypeStr=fixed  RndMeth=Round
  Complex to Real-Imag : ComplexToRealImag
  Delay24 : Delay
  Gain : Gain  Gain=sqrt(2)/2  ParamDataTypeStr=fixed  OutDataTypeStr=fixed  RndMeth=Round
  Real-Imag to Complex : RealImagToComplex
  Out1 : Outport
  wires:
  In1/1 -> Gain/1
  Real-Imag to Complex/1 -> Out1/1
  Delay24/1 -> Complex to Real-Imag/1
  Add1/1 -> Real-Imag to Complex/2
  Add/1 -> Real-Imag to Complex/1
  Complex to Real-Imag/2 -> Add/2, Add1/1
  Complex to Real-Imag/1 -> Add/1, Add1/2
  Gain/1 -> Delay24/1

== system fft_overlap_tomori/16//32 and test junk/16/FFT16/multByMinusJ ==
  x4 : Inport
  Complex to Real-Imag : ComplexToRealImag
  Real-Imag to Complex : RealImagToComplex
  Unary Minus1 : UnaryMinus
  Out1 : Outport
  wires:
  Unary Minus1/1 -> Real-Imag to Complex/2
  Real-Imag to Complex/1 -> Out1/1
  x4/1 -> Complex to Real-Imag/1
  Complex to Real-Imag/2 -> Real-Imag to Complex/1
  Complex to Real-Imag/1 -> Unary Minus1/1

== system fft_overlap_tomori/16//32 and test junk/16/FFT16/multByMinusJ3 ==
  In1 : Inport
  Complex to Real-Imag : ComplexToRealImag
  Real-Imag to Complex : RealImagToComplex
  Unary Minus1 : UnaryMinus
  Out1 : Outport
  wires:
  Unary Minus1/1 -> Real-Imag to Complex/2
  Real-Imag to Complex/1 -> Out1/1
  In1/1 -> Complex to Real-Imag/1
  Complex to Real-Imag/2 -> Real-Imag to Complex/1
  Complex to Real-Imag/1 -> Unary Minus1/1

== system fft_overlap_tomori/16//32 and test junk/16/FFT16/test ==
  In1 : Inport
  Abs1 : Abs  Commented=on  SaturateOnIntegerOverflow=off
  Abs2 : Abs  Commented=on  SaturateOnIntegerOverflow=off
  Buffer1 : Buffer  Commented=on  N=8  V=7  OutputFrames=off
  Data Type Conversion1 : DataTypeConversion  Commented=on  OutDataTypeStr=fixdt(1,16,15)  SaturateOnIntegerOverflow=off  RndMeth=Floor
  Data Type Conversion2 : DataTypeConversion  Commented=on  OutDataTypeStr=fixdt(1,16,15)  SaturateOnIntegerOverflow=off  RndMeth=Floor
  Data Type Conversion4 : DataTypeConversion  Commented=on  OutDataTypeStr=double  SaturateOnIntegerOverflow=off  RndMeth=Floor
  Data Type Conversion5 : DataTypeConversion  Commented=on  OutDataTypeStr=double  SaturateOnIntegerOverflow=off  RndMeth=Floor
  Data Type Conversion6 : DataTypeConversion  Commented=on  SaturateOnIntegerOverflow=off  RndMeth=Floor
  Delay{28..34} (7 alike) : Delay  Commented=on  DelayLength=1
  Delay35 : Delay  Commented=on  DelayLength=40
  FFT1 : dspxfrm3/FFT  Commented=on  FFTImplementation=Auto  CompMethod=Table lookup  TableOpt=NEW  TableOptActive=Speed  BitRevOrder=off  Normalize=off  InheritFFTLength=on  FFTLength=64  WrapInput=on  roundingMode=Floor  overflowMode=off  firstCoeffDataTypeStr=Inherit: Same word length as input  firstCoeffLastDataTypeStr=Inherit: Same word length as input  outputMin=[]  outputMax=[]
  Mux : Mux  Commented=on  Inputs=8
  Real-Imag to Complex : RealImagToComplex  Commented=on
  Real-Imag to Complex1 : RealImagToComplex  Commented=on
  Scope : Scope  Commented=on  NumInputPorts=2
  Scope1 : Scope  NumInputPorts=8
  Sine Wave1 : Sin  Commented=on  Frequency=2*pi*1e6  SampleTime=2e-8
  Sine Wave2 : Sin  Commented=on  Frequency=2*pi*1e6  SampleTime=2e-8
  Sine Wave3 : Sin  Commented=on  Amplitude=.99  Frequency=2*pi*1e6  Phase=pi/2  SampleTime=2e-8
  Sine Wave4 : Sin  Commented=on  Amplitude=.99  Frequency=2*pi*1e6  Phase=pi/2  SampleTime=2e-8
  Unbuffer1 : Unbuffer  Commented=on
  Unbuffer2 : Unbuffer  Commented=on
  Out1 : Outport
  wires:
  In1/1 -> Out1/1
  Delay32/1 -> Delay33/1
  Unbuffer1/1 -> Data Type Conversion4/1
  Data Type Conversion2/1 -> Data Type Conversion6/1
  Sine Wave1/1 -> Real-Imag to Complex1/2
  Delay30/1 -> Delay31/1
  Mux/1 -> Unbuffer1/1
  FFT1/1 -> Unbuffer2/1
  Data Type Conversion1/1 -> Delay28/1
  Data Type Conversion5/1 -> Abs2/1
  Data Type Conversion4/1 -> Abs1/1
  Sine Wave3/1 -> Real-Imag to Complex/1
  Delay28/1 -> Delay29/1
  Delay31/1 -> Delay32/1
  Delay29/1 -> Delay30/1
  Sine Wave4/1 -> Real-Imag to Complex1/1
  Real-Imag to Complex/1 -> Data Type Conversion2/1
  Delay35/1 -> Scope/2
  Data Type Conversion6/1 -> Buffer1/1
  Delay33/1 -> Delay34/1
  Buffer1/1 -> FFT1/1
  Abs1/1 -> Scope/1
  Sine Wave2/1 -> Real-Imag to Complex/2
  Real-Imag to Complex1/1 -> Data Type Conversion1/1
  Abs2/1 -> Delay35/1
  Unbuffer2/1 -> Data Type Conversion5/1

== system fft_overlap_tomori/16//32 and test junk/16pointfftchan1/fft_res/cmut1 ==
  In1 : Inport
  Constant : Constant  Value=s(13)  OutDataTypeStr=fixdt(1,16,15)  SampleTime=-1
  complexmult : Subsystem
  Out1 : Outport
  wires:
  Constant/1 -> complexmult/2(In3)
  complexmult/1(Out1) -> Out1/1
  In1/1 -> complexmult/1(In1)

== system fft_overlap_tomori/16//32 and test junk/16pointfftchan1/fft_res/cmut2 ==
  In1 : Inport
  Constant : Constant  Value=s(21)  OutDataTypeStr=fixdt(1,16,15)  SampleTime=-1
  complexmult : Subsystem
  Out1 : Outport
  wires:
  Constant/1 -> complexmult/2(In3)
  complexmult/1(Out1) -> Out1/1
  In1/1 -> complexmult/1(In1)

== system fft_overlap_tomori/16//32 and test junk/16pointfftchan1/fft_res/cmut21 ==
  In1 : Inport
  Constant : Constant  Value=s(5)  OutDataTypeStr=fixdt(1,16,15)  SampleTime=-1
  complexmult : Subsystem
  Out1 : Outport
  wires:
  Constant/1 -> complexmult/2(In3)
  complexmult/1(Out1) -> Out1/1
  In1/1 -> complexmult/1(In1)

== system fft_overlap_tomori/16//32 and test junk/16pointfftchan1/fft_res/cmut3 ==
  In1 : Inport
  Constant : Constant  Value=s(29)  OutDataTypeStr=fixdt(1,16,15)  SampleTime=-1
  complexmult : Subsystem
  Out1 : Outport
  wires:
  Constant/1 -> complexmult/2(In3)
  complexmult/1(Out1) -> Out1/1
  In1/1 -> complexmult/1(In1)

== system fft_overlap_tomori/16//32 and test junk/16pointfftchan1/fft_res/fft_1 ==
  In1 : Inport
  In2 : Inport  Port=2
  In3 : Inport  Port=3
  In4 : Inport  Port=4
  In5 : Inport  Port=5
  In6 : Inport  Port=6
  In7 : Inport  Port=7
  In8 : Inport  Port=8
  Add{1..3,8..9,12..13,16,18,20,22,24} (12 alike) : Sum  OutDataTypeStr=fixed_point  AccumDataTypeStr=fixed_point
  Add{4..7,10..11,14..15,17,19,21,23} (12 alike) : Sum  Inputs=+-  OutDataTypeStr=fixed_point  AccumDataTypeStr=fixed_point
  Delay{,1..15,22..26} (21 alike) : Delay  DelayLength=1
  Delay{16..20} (5 alike) : Delay  DelayLength=3
  Delay21 : Delay
  Mux : Mux  Inputs=8
  proddd : Subsystem
  ptrrt : Subsystem
  s1 : Subsystem
  s17 : Subsystem
  s2 : Subsystem
  Out1 : Outport
  wires:
  Delay26/1 -> s2/1(In1)
  Delay25/1 -> ptrrt/1(In1)
  Delay24/1 -> proddd/1(In1)
  In4/1 -> Add7/1, Add24/1
  Add15/1 -> s1/1(In1)
  Add24/1 -> Delay19/1
  In7/1 -> Add6/2, Add3/2
  Add11/1 -> s17/1(In1)
  In5/1 -> Add4/2, Add1/2
  In2/1 -> Add5/1, Add2/1
  In6/1 -> Add5/2, Add2/2
  In3/1 -> Add6/1, Add3/1
  In8/1 -> Add7/2, Add24/2
  proddd/1(Out1) -> Delay23/1
  Add2/1 -> Delay17/1
  Add3/1 -> Delay18/1
  Delay21/1 -> Add14/2, Add12/2
  In1/1 -> Add4/1, Add1/1
  Add1/1 -> Delay16/1
  ptrrt/1(Out1) -> Delay22/1
  Add17/1 -> Delay1/1
  Add18/1 -> Delay2/1
  Add19/1 -> Delay3/1
  Add20/1 -> Delay4/1
  Add21/1 -> Delay5/1
  Add22/1 -> Delay6/1
  Add23/1 -> Delay7/1
  Mux/1 -> Out1/1
  Add16/1 -> Delay/1
  Delay/1 -> Mux/1
  Delay1/1 -> Mux/2
  Delay2/1 -> Mux/3
  Delay3/1 -> Mux/4
  Delay4/1 -> Mux/5
  Delay5/1 -> Mux/6
  Delay6/1 -> Mux/7
  Delay7/1 -> Mux/8
  Add8/1 -> Delay8/1
  Add9/1 -> Delay9/1
  Add10/1 -> Delay10/1
  s17/1(Out1) -> Delay11/1
  Add12/1 -> Delay12/1
  Add13/1 -> Delay13/1
  Add14/1 -> Delay14/1
  s1/1(Out1) -> Delay15/1
  Delay16/1 -> Add10/1, Add8/1
  Delay17/1 -> Add11/1, Add9/1
  Delay18/1 -> Add10/2, Add8/2
  Delay19/1 -> Add11/2, Add9/2
  Delay20/1 -> Add14/1, Add12/1
  s2/1(Out1) -> Delay21/1
  Add5/1 -> Delay24/1
  Add6/1 -> Delay26/1
  Add7/1 -> Delay25/1
  Add4/1 -> Delay20/1
  Delay8/1 -> Add17/1, Add16/1
  Delay9/1 -> Add17/2, Add16/2
  Delay10/1 -> Add19/1, Add18/1
  Delay11/1 -> Add19/2, Add18/2
  Delay12/1 -> Add21/1, Add20/1
  Delay13/1 -> Add21/2, Add20/2
  Delay14/1 -> Add22/1, Add23/1
  Delay15/1 -> Add23/2, Add22/2
  Delay22/1 -> Add13/2, Add15/2
  Delay23/1 -> Add15/1, Add13/1

== system fft_overlap_tomori/16//32 and test junk/16pointfftchan1/fft_res/fft_8 ==
  In1 : Inport
  In2 : Inport  Port=2
  In3 : Inport  Port=3
  In4 : Inport  Port=4
  In5 : Inport  Port=5
  In6 : Inport  Port=6
  In7 : Inport  Port=7
  In8 : Inport  Port=8
  Add{1..3,8..9,12..13,16,18,20,22,24} (12 alike) : Sum  OutDataTypeStr=fixed_point  AccumDataTypeStr=fixed_point
  Add{4..7,10..11,14..15,17,19,21,23} (12 alike) : Sum  Inputs=+-  OutDataTypeStr=fixed_point  AccumDataTypeStr=fixed_point
  Delay{,1..15,22..26} (21 alike) : Delay  DelayLength=1
  Delay{16..20} (5 alike) : Delay  DelayLength=3
  Delay21 : Delay
  Mux : Mux  Inputs=8
  proddd : Subsystem
  ptrrt : Subsystem
  s1 : Subsystem
  s17 : Subsystem
  s2 : Subsystem
  Out1 : Outport
  wires:
  Delay23/1 -> Add13/1, Add15/1
  Delay22/1 -> Add15/2, Add13/2
  Delay15/1 -> Add22/2, Add23/2
  Delay14/1 -> Add23/1, Add22/1
  Delay13/1 -> Add20/2, Add21/2
  Delay12/1 -> Add20/1, Add21/1
  Delay11/1 -> Add18/2, Add19/2
  Delay10/1 -> Add18/1, Add19/1
  Delay9/1 -> Add16/2, Add17/2
  Delay8/1 -> Add16/1, Add17/1
  Add4/1 -> Delay20/1
  Add7/1 -> Delay25/1
  Add6/1 -> Delay26/1
  Add5/1 -> Delay24/1
  s2/1(Out1) -> Delay21/1
  Delay20/1 -> Add12/1, Add14/1
  Delay19/1 -> Add9/2, Add11/2
  Delay18/1 -> Add8/2, Add10/2
  Delay17/1 -> Add9/1, Add11/1
  Delay16/1 -> Add8/1, Add10/1
  s1/1(Out1) -> Delay15/1
  Add14/1 -> Delay14/1
  Add13/1 -> Delay13/1
  Add12/1 -> Delay12/1
  s17/1(Out1) -> Delay11/1
  Add10/1 -> Delay10/1
  Add9/1 -> Delay9/1
  Add8/1 -> Delay8/1
  Delay7/1 -> Mux/8
  Delay6/1 -> Mux/7
  Delay5/1 -> Mux/6
  Delay4/1 -> Mux/5
  Delay3/1 -> Mux/4
  Delay2/1 -> Mux/3
  Delay1/1 -> Mux/2
  Delay/1 -> Mux/1
  Add16/1 -> Delay/1
  Mux/1 -> Out1/1
  Add23/1 -> Delay7/1
  Add22/1 -> Delay6/1
  Add21/1 -> Delay5/1
  Add20/1 -> Delay4/1
  Add19/1 -> Delay3/1
  Add18/1 -> Delay2/1
  Add17/1 -> Delay1/1
  ptrrt/1(Out1) -> Delay22/1
  Add1/1 -> Delay16/1
  In1/1 -> Add1/1, Add4/1
  Delay21/1 -> Add12/2, Add14/2
  Add3/1 -> Delay18/1
  Add2/1 -> Delay17/1
  proddd/1(Out1) -> Delay23/1
  In8/1 -> Add24/2, Add7/2
  In3/1 -> Add3/1, Add6/1
  In6/1 -> Add2/2, Add5/2
  In2/1 -> Add2/1, Add5/1
  In5/1 -> Add1/2, Add4/2
  Add11/1 -> s17/1(In1)
  In7/1 -> Add3/2, Add6/2
  Add24/1 -> Delay19/1
  Add15/1 -> s1/1(In1)
  In4/1 -> Add24/1, Add7/1
  Delay24/1 -> proddd/1(In1)
  Delay25/1 -> ptrrt/1(In1)
  Delay26/1 -> s2/1(In1)

== system fft_overlap_tomori/16//32 and test junk/16pointfftchan1/fft_res/prod_2 ==
  In1 : Inport
  Delay24 : Delay
  Delay9 : Delay  DelayLength=1
  Gain : Gain  Gain=fi(sqrt(2)/2,1,16,15)  ParamDataTypeStr=fixdt(1,16,15)  OutDataTypeStr=fixed_point
  s3 : Subsystem
  Out1 : Outport
  wires:
  Delay9/1 -> Out1/1
  s3/1(Out1) -> Delay9/1
  In1/1 -> Gain/1
  Gain/1 -> Delay24/1
  Delay24/1 -> s3/1(In1)

== system fft_overlap_tomori/16//32 and test junk/16pointfftchan1/fft_res/prod_3 ==
  In1 : Inport
  Delay25 : Delay
  Delay9 : Delay  DelayLength=1
  Gain1 : Gain  Gain=fi(-sqrt(2)/2,1,16,15)  ParamDataTypeStr=fixdt(1,16,15)  OutDataTypeStr=fixed_point
  s4 : Subsystem
  Out1 : Outport
  wires:
  Delay9/1 -> Out1/1
  s4/1(Out1) -> Delay9/1
  In1/1 -> Gain1/1
  Delay25/1 -> s4/1(In1)
  Gain1/1 -> Delay25/1

== system fft_overlap_tomori/16//32 and test junk/16pointfftchan1/fft_res/s2 ==
  In1 : Inport
  Complex to Real-Imag : ComplexToRealImag
  Real-Imag to Complex : RealImagToComplex
  Unary Minus : UnaryMinus
  Out1 : Outport  VectorParamsAs1DForOutWhenUnconnected=off
  wires:
  In1/1 -> Complex to Real-Imag/1
  Complex to Real-Imag/2 -> Real-Imag to Complex/1
  Complex to Real-Imag/1 -> Unary Minus/1
  Unary Minus/1 -> Real-Imag to Complex/2
  Real-Imag to Complex/1 -> Out1/1
